simulink model "power_PVArray_PartialShading8"  (R2019b)
settings: Solver=ode23tb  StartTime=0.0  StopTime=3  FixedStep=Ts_Power  RelTol=1e-4
PreLoadFcn:
  | Ts_Power=50e-6;
  | Slope_Vdc=1;
InitFcn:
  | Ts_Power=50e-6;
  | Tc=1e-5;%break algebraic loop time constant
  | BlockName=[gcs,'/PV cells 1-20'];
  | ModuleName=get_param(BlockName,'ModuleName');
  | Voc1=str2num(get_param(BlockName,'Voc'));
  | Nser1=str2num(get_param(BlockName,'Nser'));
  | Slope_Vdc=Nser1*Voc1;
StopFcn:
  | if exist('I','var') && exist('V','var')
  |    figure(1)
  |    clf
  |    n=find(I>=0);
  |    n=n(end);
  |    Vglobal=V(1:n);
  |    Iglobal=I(1:n);
  | 
  | 
  |    Pglobal=Vglobal.*Iglobal;
  |    n=find(Pglobal==max(Pglobal));
  |    Pmax=Pglobal(n);
  |    Vmp=Vglobal(n);
  |    Imp=Iglobal(n);
  | 
  | 
  |    subplot(211)
  |    plot(Vglobal, Iglobal,Vmp,Imp,'or')
  |    ylabel('Current (A)')
  |    title(sprintf('Global I-V & P-V characteristics\n %s' ,ModuleName))
  | 
  | 
  |    subplot(212)
  |    plot(Vglobal, Pglobal,Vmp,Pmax,'or')
  |    ylabel('Power (W)')
  |    xlabel('Voltage (V)')
  | end
libraries: powerlib x13, re_lib x9, simulink x1
settings Model: Creator=MathWorks  LastModifiedBy=Aditya
settings SolverCC: AlgebraicLoopSolver=LineSearch
settings DataIOCC: LimitDataPoints=on  SaveFormat=Array  SignalLoggingSaveFormat=ModelDataLogs  ReturnWorkspaceOutputs=off
settings OptimizationCC: ExpressionDepthLimit=2147483647  LifeSpan=inf
settings DebuggingCC: UnderspecifiedInitializationDetection=Classic  MergeDetectMultiDrivingBlocksExec=none  SolverPrmCheckMsg=warning  FcnCallInpInsideContextMsg=warning  AllowSymbolicDim=off  StateNameClashWarn=warning  SFUnexpectedBacktrackingDiag=warning  SFNoUnconditionalDefaultTransitionDiag=warning  SFExecutionAtInitializationDiag=none  ArithmeticOperatorsInVariantConditions=warning
settings HardwareCC: ProdBitPerPointer=32  ProdBitPerSizeT=32  ProdBitPerPtrDiffT=32  ProdLargestAtomicFloat=None  ProdIntDivRoundTo=Undefined  ProdEndianess=Unspecified  ProdWordSize=32  ProdHWDeviceType=32-bit Generic
settings ModelReferenceCC: PropagateSignalLabelsOutOfModel=off
settings SFSimCC: SimUseLocalCustomCode=off  CustomCodeUndefinedFunction=UseInterfaceOnly
settings RTWCC: RTWUseLocalCustomCode=off
settings CodeAppCC: StateflowObjectComments=on
settings GRTTargetCC: TargetLangStandard=C89/C90 (ANSI)  GeneratePreprocessorConditionals=Disable all  CombineOutputUpdateFcns=off  GRTInterface=on
settings ConfigComp: CovMetricSettings=dw  CovHtmlReporting=on  CovSaveCumulativeToWorkspaceVar=on  CovSaveSingleToWorkspaceVar=on  CovExternalEMLEnable=off  CovSFcnEnable=off
settings SimscapeCC: SimscapeNormalizeSystem=off

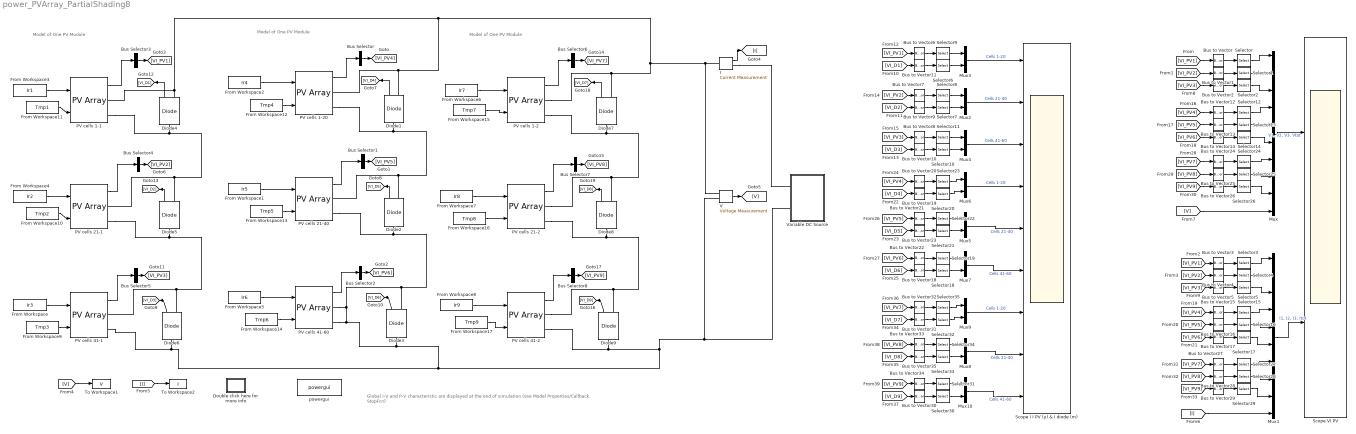
== system power_PVArray_PartialShading8 ==
  note: Global I-V and P-V characteristic are displayed at the end of simulation
      | (see Model Properties/Callback StopFcn)
  note: Model of One PV Module
  note: Model of One PV Module
  note: Model of One PV Module
  Bus Selector{,1..8} (9 alike) : BusSelector  OutputSignals=V_PV,I_PV  OutputAsBus=on
  Bus to Vector{,1..35} (36 alike) : BusToVector
  Diode{1..9} (9 alike) : powerlib/Power Electronics/Diode  Ron=0.001  Lon=0  Vf=0.7  IC=0  UseSnubber=off  Rs=1e5*inf  Cs=inf  Measurements=on
      settings: SourceProductName=Simscape Electrical
  Double click here for more info : Subsystem
      settings: OpenFcn=showdemo(bdroot(gcb))
      mask Display: disp('?')
  From Workspace : FromWorkspace  VariableName=Ir3
  From Workspace1 : FromWorkspace  VariableName=Ir5
  From Workspace10 : FromWorkspace  VariableName=Tmp2
  From Workspace11 : FromWorkspace  VariableName=Tmp1
  From Workspace12 : FromWorkspace  VariableName=Tmp4
  From Workspace13 : FromWorkspace  VariableName=Tmp5
  From Workspace14 : FromWorkspace  VariableName=Tmp6
  From Workspace15 : FromWorkspace  VariableName=Tmp7
  From Workspace16 : FromWorkspace  VariableName=Tmp8
  From Workspace17 : FromWorkspace  VariableName=Tmp9
  From Workspace2 : FromWorkspace  VariableName=Ir4
  From Workspace3 : FromWorkspace  VariableName=Ir1
  From Workspace4 : FromWorkspace  VariableName=Ir2
  From Workspace5 : FromWorkspace  VariableName=Ir6
  From Workspace6 : FromWorkspace  VariableName=Ir7
  From Workspace7 : FromWorkspace  VariableName=Ir8
  From Workspace8 : FromWorkspace  VariableName=Ir9
  From Workspace9 : FromWorkspace  VariableName=Tmp3
  I : powerlib/Measurements/Current Measurement  PhasorSimulation=off  OutputType=Complex  PSBequivalent=0
      settings: SourceProductName=Simscape Electrical
  Mux : Mux  Inputs=10
  Mux1 : Mux  Inputs=10
  Mux{2..10} (9 alike) : Mux  Inputs=2
  PV cells 1-1 : re_lib/Solar/PV Array  Npar=1  Nser=1  PlotType=array @ 25 deg.C & specified irradiances  S_vec="[ 1000  500  100 ]"  Temp_C_vec="[ 45 25  ]"  ModuleName=User-defined  PlotWhenSelected=off  Pm=83.2824  Ncell=2  Voc=37.92*20/60  Isc=8.62  Vm=30.96*20/60  Im=8.07  beta_Voc_pc=-0.33969  alpha_Isc_pc=0.063701  beta_Voc=-0.042937  alpha_Isc=0.005491  IL=9.2038  I0=1.351e-10  nI=9.8996  Rsh=14.4702  Rs=0.095042  BAL=on  Tc=Tc  Tfilter=5e-5
      settings: SourceProductName=Simscape Electrical
  PV cells 1-2 : re_lib/Solar/PV Array  Npar=1  Nser=1  PlotType=array @ 25 deg.C & specified irradiances  S_vec="[ 1000  500  100 ]"  Temp_C_vec="[ 45 25  ]"  ModuleName=User-defined  PlotWhenSelected=off  Pm=83.2824  Ncell=2  Voc=37.92*20/60  Isc=8.62  Vm=30.96*20/60  Im=8.07  beta_Voc_pc=-0.33969  alpha_Isc_pc=0.063701  beta_Voc=-0.042937  alpha_Isc=0.005491  IL=9.2038  I0=1.351e-10  nI=9.8996  Rsh=14.4702  Rs=0.095042  BAL=on  Tc=Tc  Tfilter=5e-5
      settings: SourceProductName=Simscape Electrical
  PV cells 1-20 : re_lib/Solar/PV Array  Npar=1  Nser=1  PlotType=array @ 25 deg.C & specified irradiances  S_vec="[ 1000  500  100 ]"  Temp_C_vec="[ 45 25  ]"  ModuleName=User-defined  PlotWhenSelected=off  Pm=83.2824  Ncell=2  Voc=37.92*20/60  Isc=8.62  Vm=30.96*20/60  Im=8.07  beta_Voc_pc=-0.33969  alpha_Isc_pc=0.063701  beta_Voc=-0.042937  alpha_Isc=0.005491  IL=9.2038  I0=1.351e-10  nI=9.8996  Rsh=14.4702  Rs=0.095042  BAL=on  Tc=Tc  Tfilter=5e-5
      settings: SourceProductName=Simscape Electrical
  PV cells 21-1 : re_lib/Solar/PV Array  Npar=1  Nser=1  PlotType=array @ 25 deg.C & specified irradiances  S_vec="[ 1000  500  100 ]"  Temp_C_vec="[ 45 25  ]"  ModuleName=User-defined  PlotWhenSelected=off  Pm=83.2824  Ncell=2  Voc=37.92*20/60  Isc=8.62  Vm=30.96*20/60  Im=8.07  beta_Voc_pc=-0.33969  alpha_Isc_pc=0.063701  beta_Voc=-0.042937  alpha_Isc=0.005491  IL=9.2038  I0=1.351e-10  nI=9.8996  Rsh=14.4702  Rs=0.095042  BAL=on  Tc=Tc  Tfilter=5e-5
      settings: SourceProductName=Simscape Electrical
  PV cells 21-2 : re_lib/Solar/PV Array  Npar=1  Nser=1  PlotType=array @ 25 deg.C & specified irradiances  S_vec="[ 1000  500  100 ]"  Temp_C_vec="[ 45 25  ]"  ModuleName=User-defined  PlotWhenSelected=off  Pm=83.2824  Ncell=2  Voc=37.92*20/60  Isc=8.62  Vm=30.96*20/60  Im=8.07  beta_Voc_pc=-0.33969  alpha_Isc_pc=0.063701  beta_Voc=-0.042937  alpha_Isc=0.005491  IL=9.2038  I0=1.351e-10  nI=9.8996  Rsh=14.4702  Rs=0.095042  BAL=on  Tc=Tc  Tfilter=5e-5
      settings: SourceProductName=Simscape Electrical
  PV cells 21-40 : re_lib/Solar/PV Array  Npar=1  Nser=1  PlotType=array @ 25 deg.C & specified irradiances  S_vec="[ 1000  500  100 ]"  Temp_C_vec="[ 45 25  ]"  ModuleName=User-defined  PlotWhenSelected=off  Pm=83.2824  Ncell=2  Voc=37.92*20/60  Isc=8.62  Vm=30.96*20/60  Im=8.07  beta_Voc_pc=-0.33969  alpha_Isc_pc=0.063701  beta_Voc=-0.042937  alpha_Isc=0.005491  IL=9.2038  I0=1.351e-10  nI=9.8996  Rsh=14.4702  Rs=0.095042  BAL=on  Tc=Tc  Tfilter=5e-5
      settings: SourceProductName=Simscape Electrical
  PV cells 41-1 : re_lib/Solar/PV Array  Npar=1  Nser=1  PlotType=array @ 25 deg.C & specified irradiances  S_vec="[ 1000  500  100 ]"  Temp_C_vec="[ 45 25  ]"  ModuleName=User-defined  PlotWhenSelected=off  Pm=83.2824  Ncell=2  Voc=37.92*20/60  Isc=8.62  Vm=30.96*20/60  Im=8.07  beta_Voc_pc=-0.33969  alpha_Isc_pc=0.063701  beta_Voc=-0.042937  alpha_Isc=0.005491  IL=9.2038  I0=1.351e-10  nI=9.8996  Rsh=14.4702  Rs=0.095042  BAL=on  Tc=Tc  Tfilter=5e-5
      settings: SourceProductName=Simscape Electrical
  PV cells 41-2 : re_lib/Solar/PV Array  Npar=1  Nser=1  PlotType=array @ 25 deg.C & specified irradiances  S_vec="[ 1000  500  100 ]"  Temp_C_vec="[ 45 25  ]"  ModuleName=User-defined  PlotWhenSelected=off  Pm=83.2824  Ncell=2  Voc=37.92*20/60  Isc=8.62  Vm=30.96*20/60  Im=8.07  beta_Voc_pc=-0.33969  alpha_Isc_pc=0.063701  beta_Voc=-0.042937  alpha_Isc=0.005491  IL=9.2038  I0=1.351e-10  nI=9.8996  Rsh=14.4702  Rs=0.095042  BAL=on  Tc=Tc  Tfilter=5e-5
      settings: SourceProductName=Simscape Electrical
  PV cells 41-60 : re_lib/Solar/PV Array  Npar=1  Nser=1  PlotType=array @ 25 deg.C & specified irradiances  S_vec="[ 1000  500  100 ]"  Temp_C_vec="[ 45 25  ]"  ModuleName=User-defined  PlotWhenSelected=off  Pm=83.2824  Ncell=2  Voc=37.92*20/60  Isc=8.62  Vm=30.96*20/60  Im=8.07  beta_Voc_pc=-0.33969  alpha_Isc_pc=0.063701  beta_Voc=-0.042937  alpha_Isc=0.005491  IL=9.2038  I0=1.351e-10  nI=9.8996  Rsh=14.4702  Rs=0.095042  BAL=on  Tc=Tc  Tfilter=5e-5
      settings: SourceProductName=Simscape Electrical
  Scope I I PV (y) & I diode (m) : Scope  NumInputPorts=9
  Scope VI PV : Scope  NumInputPorts=2
  Selector{,1..2,6..7,10,12..14,18,20..21,24..26,30,32..33} (18 alike) : Selector  InputPortWidth=2  IndexOptions=Index vector (dialog)  Indices=[1]  OutputSizes=1
  Selector{3..5,8..9,11,15..17,19,22..23,27..29,31,34..35} (18 alike) : Selector  InputPortWidth=2  IndexOptions=Index vector (dialog)  Indices=[2]  OutputSizes=1
  To Workspace1 : ToWorkspace  VariableName=V  SampleTime=1e-3
  To Workspace2 : ToWorkspace  VariableName=I  SampleTime=1e-3
  V : powerlib/Measurements/Voltage Measurement  PhasorSimulation=off  OutputType=Complex  PSBequivalent=0
      settings: SourceProductName=Simscape Electrical
  Variable DC Source : Subsystem
  powergui : powerlib/powergui  Priority=1  SimulationMode=Continuous  SampleTime=Ts_Power*0 + 20e-6  frequency=60  Iterations=50  frequencyindice=0  Pbase=100e6  ErrMax=1e-4  UnitsV=kV  UnitsW=MW  buscounter=0  FunctionMessages=off  echomessages=off  EnableUseOfTLC=off  CurrentSourceSwitches=on  DisableSnubberDevices=on  DisableRonSwitches=off  DisableVfSwitches=off  DisplayEquations=off  AutomaticDiscreteSolvers=off  SolverType=Tustin/Backward Euler (TBE)  Interpol=off  ExternalGateDelay=off  methode=off  Ts=0  x0status=blocks  SPID=off  SwTol=0  HookPort=off  NonlinearTolerance=1e-4  nMaxIteration=100  ContinueOnMaxIteration=off  RestoreLinks=warning  ResistiveCurrentMeasurement=off  Frange=[0:2:500]  Ylog=off  Xlog=on  ShowGrid=off  save=off  variable=ZData  structure=0  ZoomFFT=on  StartTime=0.0  cycles=1  DisplayStyle=1  fundamental=60  FreqAxis=off  MaxFrequency=1000  frequencyindicesteady=1  RmsSteady=1  display=off
      settings: SourceProductName=Simscape Electrical
  wires:
  From Workspace2/1 -> PV cells 1-20/1
  From Workspace12/1 -> PV cells 1-20/2
  From Workspace1/1 -> PV cells 21-40/1
  From Workspace13/1 -> PV cells 21-40/2
  I/1 -> [I]
  V/1 -> [V]
  From Workspace5/1 -> PV cells 41-60/1
  From Workspace14/1 -> PV cells 41-60/2
  Diode1/1 -> [VI_D4]
  Diode2/1 -> [VI_D5]
  Diode3/1 -> [VI_D6]
  PV cells 1-20/1 -> Bus Selector/1
  Bus Selector/1 -> [VI_PV4]
  Bus Selector1/1 -> [VI_PV5]
  PV cells 21-40/1 -> Bus Selector1/1
  Bus Selector2/1 -> [VI_PV6]
  PV cells 41-60/1 -> Bus Selector2/1
  Mux/1 -> Scope VI PV/1  "V1, V2, V3, Vtot"
  [VI_PV1] -> Bus to Vector/1
  [VI_PV2] -> Bus to Vector1/1
  [VI_PV3] -> Bus to Vector2/1
  Selector/1 -> Mux/1
  Selector1/1 -> Mux/2
  Selector2/1 -> Mux/3
  Mux1/1 -> Scope VI PV/2  "I1, I2, I3, Itot"
  [VI_PV1] -> Bus to Vector3/1
  [VI_PV2] -> Bus to Vector4/1
  [VI_PV3] -> Bus to Vector5/1
  Selector3/1 -> Mux1/1
  Selector4/1 -> Mux1/2
  Selector5/1 -> Mux1/3
  [VI_PV1] -> Bus to Vector6/1
  Mux3/1 -> Scope I I PV (y) & I diode (m)/1  "Cells 1-20"
  Selector9/1 -> Mux3/1
  [VI_D1] -> Bus to Vector11/1
  Selector6/1 -> Mux3/2
  [VI_PV2] -> Bus to Vector7/1
  Mux2/1 -> Scope I I PV (y) & I diode (m)/2  "Cells 21-40"
  Selector8/1 -> Mux2/1
  [VI_D2] -> Bus to Vector9/1
  Selector7/1 -> Mux2/2
  [VI_PV3] -> Bus to Vector8/1
  Mux4/1 -> Scope I I PV (y) & I diode (m)/3  "Cells 41-60"
  Selector11/1 -> Mux4/1
  [VI_D3] -> Bus to Vector10/1
  Selector10/1 -> Mux4/2
  [V] -> To Workspace1/1
  [I] -> To Workspace2/1
  Bus to Vector/1 -> Selector/1
  Bus to Vector1/1 -> Selector1/1
  Bus to Vector2/1 -> Selector2/1
  Bus to Vector3/1 -> Selector3/1
  Bus to Vector4/1 -> Selector4/1
  Bus to Vector5/1 -> Selector5/1
  Bus to Vector6/1 -> Selector9/1
  Bus to Vector7/1 -> Selector8/1
  Bus to Vector8/1 -> Selector11/1
  Bus to Vector9/1 -> Selector7/1
  Bus to Vector10/1 -> Selector10/1
  Bus to Vector11/1 -> Selector6/1
  Bus to Vector14/1 -> Selector14/1
  Bus to Vector13/1 -> Selector13/1
  Bus to Vector12/1 -> Selector12/1
  [VI_PV6] -> Bus to Vector14/1
  [VI_PV5] -> Bus to Vector13/1
  [VI_PV4] -> Bus to Vector12/1
  Selector14/1 -> Mux/6
  Selector13/1 -> Mux/5
  Selector12/1 -> Mux/4
  [VI_PV4] -> Bus to Vector15/1
  Bus to Vector15/1 -> Selector15/1
  [VI_PV6] -> Bus to Vector17/1
  Selector17/1 -> Mux1/6
  [VI_PV5] -> Bus to Vector16/1
  Bus to Vector17/1 -> Selector17/1
  Selector16/1 -> Mux1/5
  Selector15/1 -> Mux1/4
  Bus to Vector16/1 -> Selector16/1
  Bus to Vector19/1 -> Selector20/1
  Bus to Vector23/1 -> Selector21/1
  Bus to Vector22/1 -> Selector19/1
  [VI_D6] -> Bus to Vector18/1
  Bus to Vector21/1 -> Selector22/1
  [VI_D5] -> Bus to Vector23/1
  Selector22/1 -> Mux5/1
  Selector18/1 -> Mux7/2
  Selector19/1 -> Mux7/1
  Selector20/1 -> Mux6/2
  Selector21/1 -> Mux5/2
  [VI_PV6] -> Bus to Vector22/1
  Mux7/1 -> Scope I I PV (y) & I diode (m)/6  "Cells 41-60"
  Bus to Vector20/1 -> Selector23/1
  Mux6/1 -> Scope I I PV (y) & I diode (m)/4  "Cells 1-20"
  [VI_D4] -> Bus to Vector19/1
  Mux5/1 -> Scope I I PV (y) & I diode (m)/5  "Cells 21-40"
  Selector23/1 -> Mux6/1
  [VI_PV4] -> Bus to Vector20/1
  [VI_PV5] -> Bus to Vector21/1
  Bus to Vector18/1 -> Selector18/1
  From Workspace10/1 -> PV cells 21-1/2
  Diode4/1 -> [VI_D1]
  From Workspace11/1 -> PV cells 1-1/2
  From Workspace9/1 -> PV cells 41-1/2
  Bus Selector4/1 -> [VI_PV2]
  Bus Selector3/1 -> [VI_PV1]
  PV cells 41-1/1 -> Bus Selector5/1
  Diode6/1 -> [VI_D3]
  Bus Selector5/1 -> [VI_PV3]
  PV cells 1-1/1 -> Bus Selector3/1
  Diode5/1 -> [VI_D2]
  PV cells 21-1/1 -> Bus Selector4/1
  From Workspace3/1 -> PV cells 1-1/1
  [V] -> Mux/10
  [VI_PV8] -> Bus to Vector25/1
  [VI_PV9] -> Bus to Vector26/1
  Bus to Vector24/1 -> Selector24/1
  Bus to Vector25/1 -> Selector25/1
  [VI_PV7] -> Bus to Vector24/1
  Bus to Vector26/1 -> Selector26/1
  Selector24/1 -> Mux/7
  Selector25/1 -> Mux/8
  Selector26/1 -> Mux/9
  [I] -> Mux1/10
  Selector28/1 -> Mux1/8
  Selector29/1 -> Mux1/9
  Bus to Vector29/1 -> Selector29/1
  [VI_PV7] -> Bus to Vector27/1
  [VI_PV9] -> Bus to Vector29/1
  Bus to Vector27/1 -> Selector27/1
  [VI_PV8] -> Bus to Vector28/1
  Selector27/1 -> Mux1/7
  Bus to Vector28/1 -> Selector28/1
  Mux8/1 -> Scope I I PV (y) & I diode (m)/8  "Cells 21-40"
  Mux10/1 -> Scope I I PV (y) & I diode (m)/9  "Cells 41-60"
  Bus to Vector30/1 -> Selector30/1
  [VI_PV8] -> Bus to Vector33/1
  [VI_PV7] -> Bus to Vector32/1
  [VI_D7] -> Bus to Vector31/1
  Mux9/1 -> Scope I I PV (y) & I diode (m)/7  "Cells 1-20"
  Selector35/1 -> Mux9/1
  Bus to Vector32/1 -> Selector35/1
  Selector33/1 -> Mux8/2
  Selector32/1 -> Mux9/2
  [VI_PV9] -> Bus to Vector34/1
  Selector34/1 -> Mux8/1
  Bus to Vector33/1 -> Selector34/1
  Selector30/1 -> Mux10/2
  [VI_D8] -> Bus to Vector35/1
  Selector31/1 -> Mux10/1
  Bus to Vector34/1 -> Selector31/1
  Bus to Vector35/1 -> Selector33/1
  [VI_D9] -> Bus to Vector30/1
  Bus to Vector31/1 -> Selector32/1
  From Workspace16/1 -> PV cells 21-2/2
  Diode7/1 -> [VI_D7]
  From Workspace15/1 -> PV cells 1-2/2
  From Workspace17/1 -> PV cells 41-2/2
  Bus Selector7/1 -> [VI_PV8]
  Bus Selector6/1 -> [VI_PV7]
  PV cells 41-2/1 -> Bus Selector8/1
  Diode9/1 -> [VI_D9]
  Bus Selector8/1 -> [VI_PV9]
  PV cells 1-2/1 -> Bus Selector6/1
  Diode8/1 -> [VI_D8]
  From Workspace7/1 -> PV cells 21-2/1
  PV cells 21-2/1 -> Bus Selector7/1
  From Workspace6/1 -> PV cells 1-2/1
  From Workspace/1 -> PV cells 41-1/1
  From Workspace4/1 -> PV cells 21-1/1
  From Workspace8/1 -> PV cells 41-2/1
  connections:
  I/RConn1 -- Variable DC Source/LConn1
  Diode6/RConn1 -- PV cells 41-1/RConn1 -- PV cells 21-1/RConn2 -- Diode5/LConn1
  Diode9/RConn1 -- Diode8/LConn1 -- PV cells 21-2/RConn2 -- PV cells 41-2/RConn1
  Diode7/LConn1 -- PV cells 21-2/RConn1 -- Diode8/RConn1 -- PV cells 1-2/RConn2
  PV cells 21-1/RConn1 -- Diode5/RConn1 -- PV cells 1-1/RConn2 -- Diode4/LConn1
  Diode2/LConn1 -- PV cells 21-40/RConn2 -- PV cells 41-60/RConn1 -- Diode9/LConn1 -- PV cells 41-2/RConn2 -- Variable DC Source/LConn2 -- V/LConn2 -- PV cells 41-1/RConn2 -- Diode6/LConn1 -- Diode3/LConn1 -- PV cells 41-60/RConn2 -- Diode3/RConn1
  PV cells 1-1/RConn1 -- PV cells 1-2/RConn1 -- Diode7/RConn1 -- V/LConn1 -- I/LConn1 -- PV cells 1-20/RConn1 -- Diode1/RConn1 -- Diode4/RConn1
  PV cells 1-20/RConn2 -- PV cells 21-40/RConn1 -- Diode2/RConn1 -- Diode1/LConn1

== system power_PVArray_PartialShading8/Double click here for more info ==

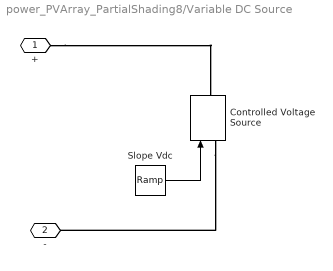
== system power_PVArray_PartialShading8/Variable DC Source ==
  Controlled Voltage Source : powerlib/Electrical Sources/Controlled Voltage Source  Initialize=on  Source_Type=AC  Amplitude=0  Phase=0  Frequency=0  Measurements=None
      settings: SourceProductName=Simscape Electrical
  Slope Vdc : simulink/Sources/Ramp  slope=Slope_Vdc  start=0  InitialOutput=0
  + : PMIOPort  Side=Left
  - : PMIOPort  Port=2  Side=Left
  wires:
  Slope Vdc/1 -> Controlled Voltage Source/1
  connections:
  Controlled Voltage Source/LConn1 -- -/RConn1
  +/RConn1 -- Controlled Voltage Source/RConn1
